simulink model "psbbreaker"  (Simulink 6.0)
settings: Solver=ode23tb  SolverMode=SingleTasking  StartTime=0.0  StopTime=0.1  MaxStep=100e-6  RelTol=1e-3
libraries: powerlib2 x6, powerlib_extras x1
settings Model: Creator=patrice  LastModifiedBy=batserve  ExtModeTrigMode=oneshot  ExtModeArmWhenConnect=off  ExtModeAutoUpdateStatusClock=off
settings DataIOCC: LimitDataPoints=off  SignalLoggingName=sigsOut
settings OptimizationCC: BooleanDataType=off
settings DebuggingCC: SolverPrmCheckMsg=none
settings HardwareCC: TargetUnknown=on
settings RTWCC: TemplateMakefile=grt_unix.tmf

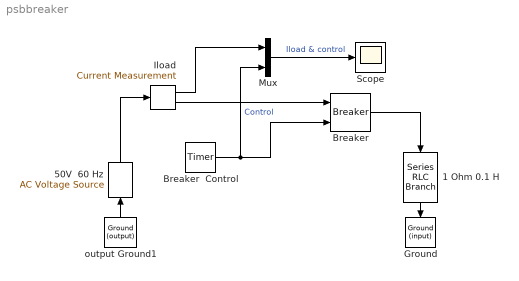
== system psbbreaker ==
  1 Ohm 0.1 H : powerlib2/Elements/Series RLC Branch  Tag=PoWeRsYsTeMbLoCk  Orientation=down  a=1  b=0.1  c=inf  mesure=None  PSBOutputType=1
  50V  60 Hz : powerlib2/Electrical Sources/AC Voltage Source  Tag=PoWeRsYsTeMbLoCk  Orientation=up  A=50  P=0  F=60  stime=0  mesure=None  PSBOutputType=1
  Breaker : powerlib2/Elements/Breaker  Tag=PoWeRsYsTeMbLoCk  a=1e-4  c=1  rs=1e6  cs=inf  times="[ 4/60  5/60 ]"  Ts=0  comext=on  mesure=None  PSBOutputType=1
  Breaker  Control : powerlib_extras/Control  Blocks/Timer  t=[0 1.5/60 3/60]  e=[1 0 1 ]
  Ground : powerlib2/Connectors/Ground (input)  Tag=PoWeRsYsTeMbLoCk  Orientation=down
  Iload : powerlib2/Measurements/Current Measurement  Tag=PoWeRsYsTeMmEaSuReMeNt  PhasorSimulation=off  OutputType=Magnitude  PSBOutputType=01  PSBequivalent=0
  Mux : Mux  Inputs=2
  Scope : Scope
      settings: TimeRange=0.1  YMin=-2  YMax=3  DataFormat=Array
  output Ground1 : powerlib2/Connectors/Ground (output)  Tag=PoWeRsYsTeMbLoCk  Orientation=up  PSBOutputType=1
  wires:
  Iload/2 -> Breaker/1
  Mux/1 -> Scope/1  "Iload & control"
  Iload/1 -> Mux/1
  50V  60 Hz/1 -> Iload/1
  output Ground1/1 -> 50V  60 Hz/1
  1 Ohm 0.1 H/1 -> Ground/1
  Breaker/1 -> 1 Ohm 0.1 H/1
  Breaker  Control/1 -> Breaker/2, Mux/2  "Control"
